simulink library "UMNBlocks_Lib"  (R2016b)
settings: Solver=VariableStepAuto  StartTime=0.0  StopTime=10.0  RelTol=1e-3
libraries: simulink x1
settings Model: Creator=UAVLAB  LastModifiedBy=UAVLAB

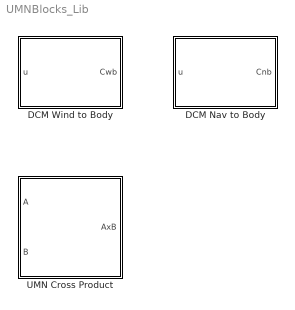
== system UMNBlocks_Lib ==
  DCM Nav to Body : MATLAB Function  TreatAsAtomicUnit=on
  DCM Wind to Body : MATLAB Function  TreatAsAtomicUnit=on
  UMN Cross Product : Subsystem

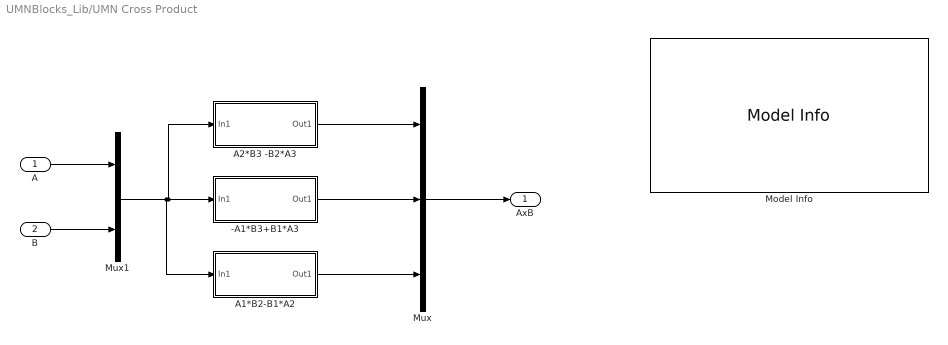
== system UMNBlocks_Lib/UMN Cross Product ==
  A : Inport
  B : Inport  Port=2
  -A1*B3+B1*A3 : Subsystem
  A1*B2-B1*A2 : Subsystem
  A2*B3 -B2*A3 : Subsystem
  Model Info : simulink/Model-Wide Utilities/Model Info  Frame=off  DisplayStringWithTags=|  HorizontalTextAlignment=Left  LeftAlignmentValue=0.02  SourceBlockDiagram=UMNBlocks_Lib  TagMaxNumber=20
      | [     i          j        k      ]
      | [   A1      A2      A3     ]
      | [   B1      B2      B3    ]
  Mux : Mux  Inputs=3
  Mux1 : Mux  Inputs=2
  AxB : Outport
  wires:
  A1*B2-B1*A2/1(Out1) -> Mux/3
  A/1 -> Mux1/1
  B/1 -> Mux1/2
  Mux/1 -> AxB/1
  -A1*B3+B1*A3/1(Out1) -> Mux/2
  A2*B3 -B2*A3/1(Out1) -> Mux/1
  Mux1/1 -> A2*B3 -B2*A3/1(In1), -A1*B3+B1*A3/1(In1), A1*B2-B1*A2/1(In1)

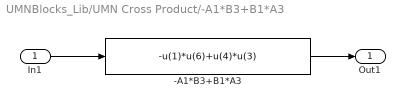
== system UMNBlocks_Lib/UMN Cross Product/-A1*B3+B1*A3 ==
  In1 : Inport
  -A1*B3+B1*A3 : Fcn  Expr=-u(1)*u(6)+u(4)*u(3)
  Out1 : Outport
  wires:
  -A1*B3+B1*A3/1 -> Out1/1
  In1/1 -> -A1*B3+B1*A3/1

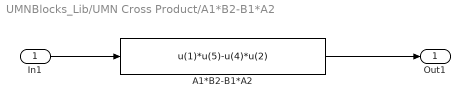
== system UMNBlocks_Lib/UMN Cross Product/A1*B2-B1*A2 ==
  In1 : Inport
  A1*B2-B1*A2 : Fcn  Expr=u(1)*u(5)-u(4)*u(2)
  Out1 : Outport
  wires:
  A1*B2-B1*A2/1 -> Out1/1
  In1/1 -> A1*B2-B1*A2/1

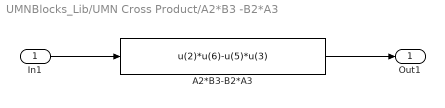
== system UMNBlocks_Lib/UMN Cross Product/A2*B3 -B2*A3 ==
  In1 : Inport
  A2*B3-B2*A3 : Fcn  Expr=u(2)*u(6)-u(5)*u(3)
  Out1 : Outport
  wires:
  A2*B3-B2*A3/1 -> Out1/1
  In1/1 -> A2*B3-B2*A3/1

== matlab function UMNBlocks_Lib/DCM Wind to Body ==
  data: u input; Cwb output
function Cwb = Simulink_ab2Cwb(u)

%% ALPHA BETA FROM WIND TO BODY
PSI_nb = -1*[0 -u(1) u(2)] ; % had to switch signs?



%% FROM NAV TO BODY
C1 = [  1               0           0           ;...
        0       cos(PSI_nb(1))  sin(PSI_nb(1))  ;...
        0       -sin(PSI_nb(1)) cos(PSI_nb(1))] ;
    
C2 = [  cos(PSI_nb(2))      0       -sin(PSI_nb(2)) ;...
            0               1           0           ;...
        sin(PSI_nb(2))      0       cos(PSI_nb(2))] ;
    
C3 = [  cos(PSI_nb(3))      sin(PSI_nb(3))      0       ;...
        -sin(PSI_nb(3))     cos(PSI_nb(3))      0       ;...
                0               0               1]      ;
         
Cnb = (C1*C2*C3);


%% FROM BODY TO NAV
Cbn = Cnb' ;


%% FROM WIND TO BODY
Cwb = Cbn' ;


end

== matlab function UMNBlocks_Lib/DCM Nav to Body ==
  data: u input; Cnb output
function Cnb = Simulink_eul2Cnb(u)

% 3 2 1 angles
PSI_nb = [u(3) u(2) u(1)];



%% FROM NAV TO BODY
C1 = [  1               0           0           ;...
        0       cos(PSI_nb(1))  sin(PSI_nb(1))  ;...
        0       -sin(PSI_nb(1)) cos(PSI_nb(1))] ;
    
C2 = [  cos(PSI_nb(2))      0       -sin(PSI_nb(2)) ;...
            0               1           0           ;...
        sin(PSI_nb(2))      0       cos(PSI_nb(2))] ;
    
C3 = [  cos(PSI_nb(3))      sin(PSI_nb(3))      0       ;...
        -sin(PSI_nb(3))     cos(PSI_nb(3))      0       ;...
                0               0               1]      ;
         
Cnb = (C1*C2*C3);


end
